simulink model "TST_AdvancedStateflowLoops2"  (Simulink 10.0)
settings: Solver=FixedStepDiscrete  StartTime=0.0  StopTime=10.0  FixedStep=0.02  RelTol=1e-3  EnableMultiTasking=on
settings Model: Creator=kharthforeign  LastModifiedBy=unknown
settings DataIOCC: LimitDataPoints=on  SignalLoggingSaveFormat=ModelDataLogs  SaveOutput=off  SignalLogging=off  SaveTime=off
settings OptimizationCC: BlockReduction=off  ConditionallyExecuteInputs=off  OptimizeBlockIOStorage=off  BufferReuse=off  GlobalBufferReuse=off  ExpressionFolding=off  ExpressionDepthLimit=2147483647  LocalBlockOutputs=off  InitFltsAndDblsToZero=on  OptimizeDataStoreBuffers=off  BusAssignmentInplaceUpdate=off
settings DebuggingCC: SolverPrmCheckMsg=warning  FcnCallInpInsideContextMsg=warning  StateNameClashWarn=warning
settings SFSimCC: SimParseCustomCode=off
settings GRTTargetCC: GeneratePreprocessorConditionals=Disable all
settings ConfigComp: CovExternalEMLEnable=off

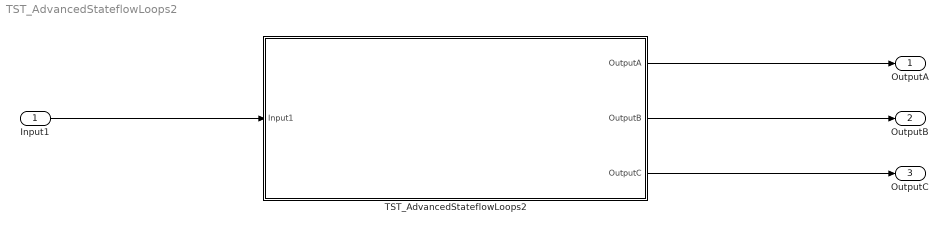
== system TST_AdvancedStateflowLoops2 ==
  Input1 : Inport  OutDataTypeStr=uint32  BusOutputAsStruct=on
  TST_AdvancedStateflowLoops2 : Subsystem  TreatAsAtomicUnit=on
  OutputA : Outport  OutDataTypeStr=double  PortDimensions=1
  OutputB : Outport  Port=2  OutDataTypeStr=double  PortDimensions=1
  OutputC : Outport  Port=3  OutDataTypeStr=double  PortDimensions=1
  wires:
  Input1/1 -> TST_AdvancedStateflowLoops2/1(Input1)
  TST_AdvancedStateflowLoops2/1(OutputA) -> OutputA/1
  TST_AdvancedStateflowLoops2/2(OutputB) -> OutputB/1
  TST_AdvancedStateflowLoops2/3(OutputC) -> OutputC/1

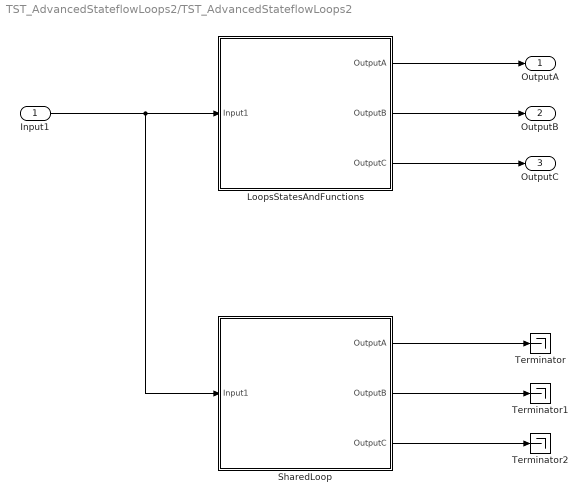
== system TST_AdvancedStateflowLoops2/TST_AdvancedStateflowLoops2 ==
  Input1 : Inport  OutDataTypeStr=uint32  BusOutputAsStruct=on
  LoopsStatesAndFunctions : Stateflow chart  TreatAsAtomicUnit=on
  SharedLoop : Stateflow chart  TreatAsAtomicUnit=on
  Terminator : Terminator
  Terminator1 : Terminator
  Terminator2 : Terminator
  OutputA : Outport  OutDataTypeStr=double  PortDimensions=1
  OutputB : Outport  Port=2  OutDataTypeStr=double  PortDimensions=1
  OutputC : Outport  Port=3  OutDataTypeStr=double  PortDimensions=1
  wires:
  LoopsStatesAndFunctions/1(OutputA) -> OutputA/1
  LoopsStatesAndFunctions/2(OutputB) -> OutputB/1
  LoopsStatesAndFunctions/3(OutputC) -> OutputC/1
  Input1/1 -> LoopsStatesAndFunctions/1(Input1), SharedLoop/1(Input1)
  SharedLoop/1(OutputA) -> Terminator/1
  SharedLoop/2(OutputB) -> Terminator1/1
  SharedLoop/3(OutputC) -> Terminator2/1

== stateflow chart TST_AdvancedStateflowLoops2/LoopsStatesAndFunctions ==
  state Ping
  state Pong
    state PongSubA
    state PongSubB
    note: demonstrate a loop inside a state
    (default) -> (junction 11)
    (junction 11) -> (junction 11) [order 1] : [C]{OutputC = 5.0;}
    (junction 11) -> PongSubA [order 2]
    PongSubA -> PongSubB : [Iterate(uint32(3))]
    PongSubB -> PongSubA : [Iterate(uint32(4))]
  state x = Iterate(b) [function]
    note: demonstrate a loop instide a function
    (default) -> (junction 20) : {Count = uint32(0);}
    (junction 20) -> (junction 21) [order 2] : {x = true;}
    (junction 22) -> (junction 20) : {OutputC = ...
        | OutputC * OutputC;}
    (junction 20) -> (junction 22) [order 1] : [Count < b]...
        | {Count += uint32(1);}
  note: demonstrate a loop between states
  (default) -> Ping
  Ping -> Pong [order 1] : [A]{OutputA = 2.0;}
  Ping -> (junction 35) [order 2]
  (junction 35) -> Pong [order 2]
  (junction 35) -> (junction 36) [order 1] : [B]{OutputB = 3.0;}
  (junction 36) -> (junction 35) : {OutputB += 1.0;}
  data: Count temporary uint32; b function_input uint32; x function_output boolean; Input1 input uint32; OutputA output double =1; OutputB output double =2; OutputC output double =3; Local local uint32 =0; A local boolean; B local boolean; C local boolean

== stateflow chart TST_AdvancedStateflowLoops2/SharedLoop ==
  state StateA
  state StateB
  state StateC
  note: demonstrate a flowgraph-loop on a joined path
      | with two different sources
  (default) -> StateA
  StateA -> StateB [order 1] : [Input1 > 5]
  StateA -> (junction 58) [order 2]
  StateB -> (junction 58) : [Input1 < 5]
  (junction 58) -> (junction 59) : [A]
  (junction 59) -> StateC [order 2] : /{OutputC = 7.0}
  (junction 61) -> (junction 59) : {OutputB += 2.0}
  (junction 59) -> (junction 60) [order 1] : [B]
  (junction 60) -> (junction 61)
  data: Input1 input uint32; OutputA output double =1; OutputB output double =2; OutputC output double =3; Local local uint32 =0; A local boolean; B local boolean; C local boolean; D local boolean
